simulink model "Planta_lineal"  (R2022a)
settings: Solver=VariableStepAuto  StartTime=0.0  StopTime=10.0  RelTol=1e-3
undefined symbols (not defined in the file): g, Ix, Iy, Iz, m, Pr
libraries: simulink x9
settings Model: Creator=juani  LastModifiedBy=juani

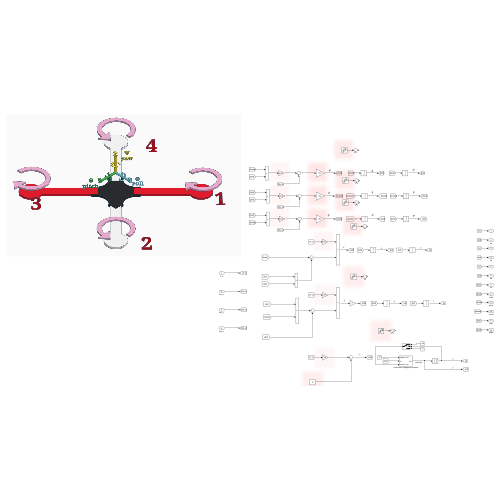
[thumbnail: Simulink's stored preview of the top-level diagram]
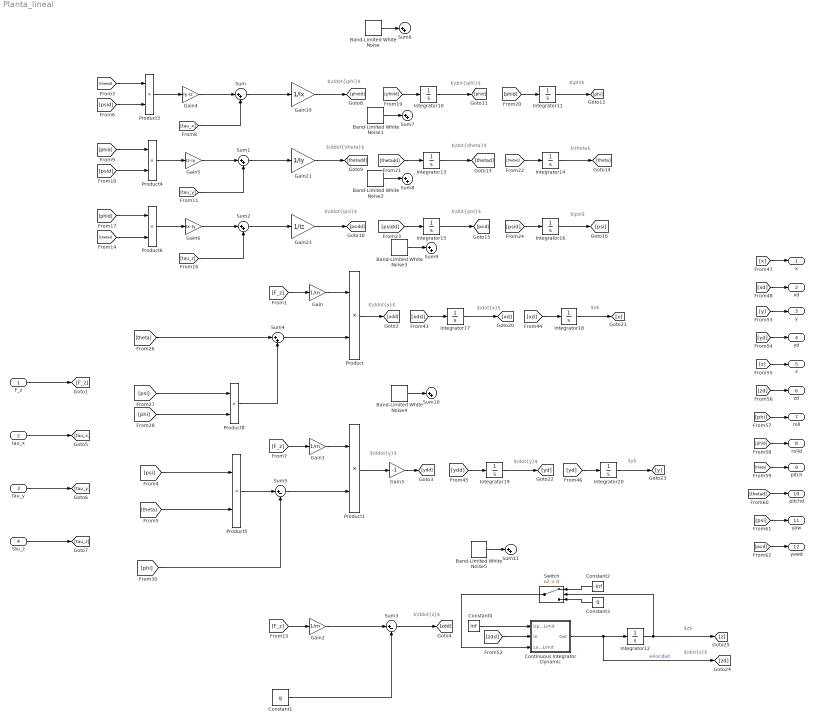
== system Planta_lineal ==
  note: $\ddot{\theta}$
  note: $\dot{\phi}$
  note: $\ddot{\phi}$
  note: $x$
  note: $\dot{\theta}$
  note: $\phi$
  note: $\theta$
  note: $\psi$
  note: $\dot{\psi}$
  note: $\ddot{x}$
  note: $\ddot{y}$
  note: $\dot{x}$
  note: $\dot{z}$
  note: $y$
  note: $\dot{y}$
  note: $z$
  note: $\ddot{z}$
  note: $\ddot{\psi}$
  F_z : Inport
  tau_x : Inport  Port=2
  tau_y : Inport  Port=3
  tau_z : Inport  Port=4
  Band-Limited White Noise{,1..5} (6 alike) : simulink/Sources/Band-Limited White Noise  Cov=[Pr]  Ts=0.1  seed=[23341]
  Constant1 : Constant  Value=g
  Constant2 : Constant  Value=-inf
  Constant3 : Constant  Value=0
  Constant4 : Constant  Value=inf
  Continuous Integrator Dynamic : Subsystem
  Gain : Gain  Gain=1/m
  Gain1 : Gain  Gain=1/m
  Gain19 : Gain  Gain=1/Ix
  Gain2 : Gain  Gain=1/m
  Gain21 : Gain  Gain=1/Iy
  Gain23 : Gain  Gain=1/Iz
  Gain3 : Gain  Gain=-1
  Gain4 : Gain  Gain=Iy-Iz
  Gain5 : Gain  Gain=Iz-Ix
  Gain6 : Gain  Gain=Ix-Iy
  Integrator{10..11,13..20} (10 alike) : Integrator
  Integrator12 : Integrator  LimitOutput=on  LowerSaturationLimit=0
  Product{,1,3..6,8} (7 alike) : Product
  Sum{,1..2,4,6..11} (10 alike) : Sum  Inputs=|++
  Sum3 : Sum  Inputs=|+-
  Sum5 : Sum  Inputs=|+-
  Switch : Switch  Criteria=u2 > Threshold  SaturateOnIntegerOverflow=off  InputSameDT=off
  x : Outport
  xd : Outport  Port=2
  y : Outport  Port=3
  yd : Outport  Port=4
  z : Outport  Port=5
  zd : Outport  Port=6
  roll : Outport  Port=7
  rolld : Outport  Port=8
  pitch : Outport  Port=9
  pitchd : Outport  Port=10
  yaw : Outport  Port=11
  yawd : Outport  Port=12
  wires:
  [phid] -> Product4/1
  Product1/1 -> Gain3/1
  [phid] -> Integrator11/1
  Integrator16/1 -> [psi]
  [phid] -> Product6/1
  Gain2/1 -> Sum3/1
  [thetad] -> Product3/1
  Product6/1 -> Gain6/1
  [psid] -> yawd/1
  Constant3/1 -> Switch/3
  Sum1/1 -> Gain21/1
  Gain4/1 -> Sum/1
  Gain6/1 -> Sum2/1
  [tau_x] -> Sum/2
  Sum4/1 -> Product/2
  Sum3/1 -> [zdd]
  Gain19/1 -> [phidd]
  Sum/1 -> Gain19/1
  [F_z] -> Gain2/1
  Gain/1 -> Product/1
  Product4/1 -> Gain5/1
  [theta] -> pitch/1
  [phid] -> rolld/1
  [phi] -> roll/1
  [z] -> z/1
  [yd] -> yd/1
  Integrator19/1 -> [yd]
  [xd] -> xd/1
  [yd] -> Integrator20/1
  tau_y/1 -> [tau_y]
  tau_x/1 -> [tau_x]
  [psi] -> yaw/1
  [psidd] -> Integrator15/1
  Integrator11/1 -> [phi]
  Band-Limited White Noise4/1 -> Sum10/1
  Band-Limited White Noise2/1 -> Sum8/1
  Band-Limited White Noise3/1 -> Sum9/1
  Sum5/1 -> Product1/2
  Gain5/1 -> Sum1/1
  [tau_z] -> Sum2/2
  [theta] -> Product5/2
  [psid] -> Product3/2
  Band-Limited White Noise1/1 -> Sum7/1
  Integrator17/1 -> [xd]
  Gain21/1 -> [thetadd]
  tau_z/1 -> [tau_z]
  F_z/1 -> [F_z]
  Integrator20/1 -> [y]
  [zd] -> zd/1
  [psid] -> Integrator16/1
  Integrator13/1 -> [thetad]
  Switch/1 -> Continuous Integrator Dynamic/3(Lower Limit)
  [thetad] -> Integrator14/1
  Product/1 -> [xdd]
  [zdd] -> Continuous Integrator Dynamic/2(In)
  [xd] -> Integrator18/1
  Integrator18/1 -> [x]
  Product5/1 -> Sum5/1
  [phidd] -> Integrator10/1
  [xdd] -> Integrator17/1
  Constant1/1 -> Sum3/2
  Gain3/1 -> [ydd]
  Integrator12/1 -> [z], Switch/2
  [tau_y] -> Sum1/2
  Product8/1 -> Sum4/2
  [ydd] -> Integrator19/1
  Band-Limited White Noise5/1 -> Sum11/1
  Product3/1 -> Gain4/1
  [psid] -> Product4/2
  [y] -> y/1
  [psi] -> Product8/1
  Integrator15/1 -> [psid]
  [phi] -> Product8/2
  [x] -> x/1
  [theta] -> Sum4/1
  Constant4/1 -> Continuous Integrator Dynamic/1(Upper Limit)
  Constant2/1 -> Switch/1
  [thetadd] -> Integrator13/1
  [thetad] -> pitchd/1
  Integrator10/1 -> [phid]
  Integrator14/1 -> [theta]
  [thetad] -> Product6/2
  Sum2/1 -> Gain23/1
  Gain23/1 -> [psidd]
  [F_z] -> Gain1/1
  [F_z] -> Gain/1
  Band-Limited White Noise/1 -> Sum6/1
  Continuous Integrator Dynamic/1(Out) -> [zd], Integrator12/1  "velocidad"
  Gain1/1 -> Product1/1
  [phi] -> Sum5/2
  [psi] -> Product5/1

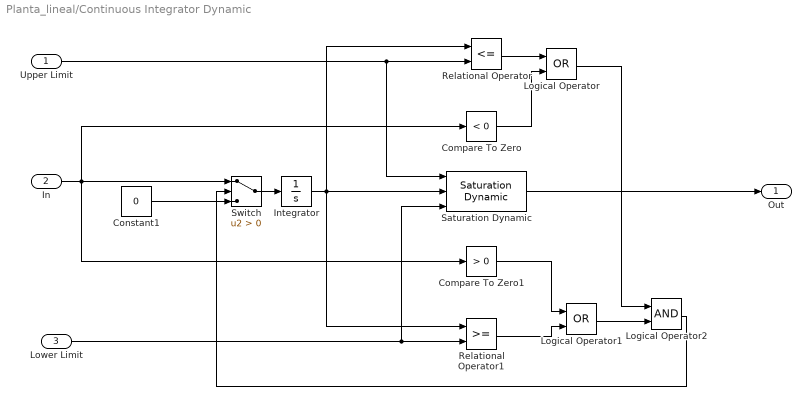
== system Planta_lineal/Continuous Integrator Dynamic ==
  Upper Limit : Inport
  In : Inport  Port=2
  Lower Limit : Inport  Port=3
  Compare To Zero : simulink/Logic and Bit Operations/Compare To Zero  relop=<  OutDataTypeStr=uint8  ZeroCross=off
  Compare To Zero1 : simulink/Logic and Bit Operations/Compare To Zero  relop=>  OutDataTypeStr=uint8  ZeroCross=off
  Constant1 : Constant  Value=0
  Integrator : Integrator
  Logical Operator : Logic  Operator=OR  AllPortsSameDT=off  OutDataTypeStr=boolean
  Logical Operator1 : Logic  Operator=OR  AllPortsSameDT=off  OutDataTypeStr=boolean
  Logical Operator2 : Logic  AllPortsSameDT=off  OutDataTypeStr=boolean
  Relational Operator : RelationalOperator  Operator=<=  OutDataTypeStr=boolean  InputSameDT=off
  Relational Operator1 : RelationalOperator  OutDataTypeStr=boolean  InputSameDT=off
  Saturation Dynamic : simulink/Discontinuities/Saturation Dynamic  OutMin=[]  OutMax=[]  OutDataTypeStr=Inherit: Same as second input  OutDataType=fixdt(1, 16)  OutScaling=2^-10  DoSatur=off
  Switch : Switch  Criteria=u2 > Threshold  SaturateOnIntegerOverflow=off  InputSameDT=off
  Out : Outport  VectorParamsAs1DForOutWhenUnconnected=off
  wires:
  In/1 -> Compare To Zero/1, Compare To Zero1/1, Switch/1
  Constant1/1 -> Switch/3
  Switch/1 -> Integrator/1
  Relational Operator/1 -> Logical Operator/1
  Compare To Zero/1 -> Logical Operator/2
  Upper Limit/1 -> Relational Operator/2, Saturation Dynamic/1
  Lower Limit/1 -> Relational Operator1/2, Saturation Dynamic/3
  Compare To Zero1/1 -> Logical Operator1/1
  Relational Operator1/1 -> Logical Operator1/2
  Logical Operator1/1 -> Logical Operator2/2
  Logical Operator/1 -> Logical Operator2/1
  Logical Operator2/1 -> Switch/2
  Saturation Dynamic/1 -> Out/1
  Integrator/1 -> Relational Operator/1, Relational Operator1/1, Saturation Dynamic/2
